simulink model "IP_SwingUp_Design21"  (R2021a)
settings: Solver=VariableStepAuto  StartTime=0.0  StopTime=30  FixedStep=0.01  RelTol=1e-3
values from neighbouring files (symbols this model uses):
  b = 0.0    (= 0)    [Init_Setup_LQRArd.m]
  c = 1.5    [Init_Setup_LQRArd.m]
  Er = 2*m*g*l    (= 0.36113784)    [Init_Setup_LQRArd.m]
  g = 9.8    [Init_Setup_LQRArd.m]
  I = 0.00527    [Init_Setup_LQRArd.m]
  l = 0.26322    [Init_Setup_LQRArd.m]
  M = 0.25    [Init_Setup_LQRArd.m]
  m = 0.07    [Init_Setup_LQRArd.m]
  M_c = 0.25    [Init_Setup_LQRArd.m]
  n = 1.05    [Init_Setup_LQRArd.m]
libraries: simulink x4
settings Model: Creator=jitendra  LastModifiedBy=M7540
settings SolverCC: AlgebraicLoopSolver=LineSearch
settings DataIOCC: ExternalInput=getinputstruct(op_trim1)  InitialState=getstatestruct(op_trim1)  ReturnWorkspaceOutputs=off
settings DebuggingCC: SFMachineParentedDataDiag=warning  ArithmeticOperatorsInVariantConditions=warning
settings SFSimCC: SimUseLocalCustomCode=off  CustomCodeUndefinedFunction=UseInterfaceOnly
settings RTWCC: RTWUseLocalCustomCode=off

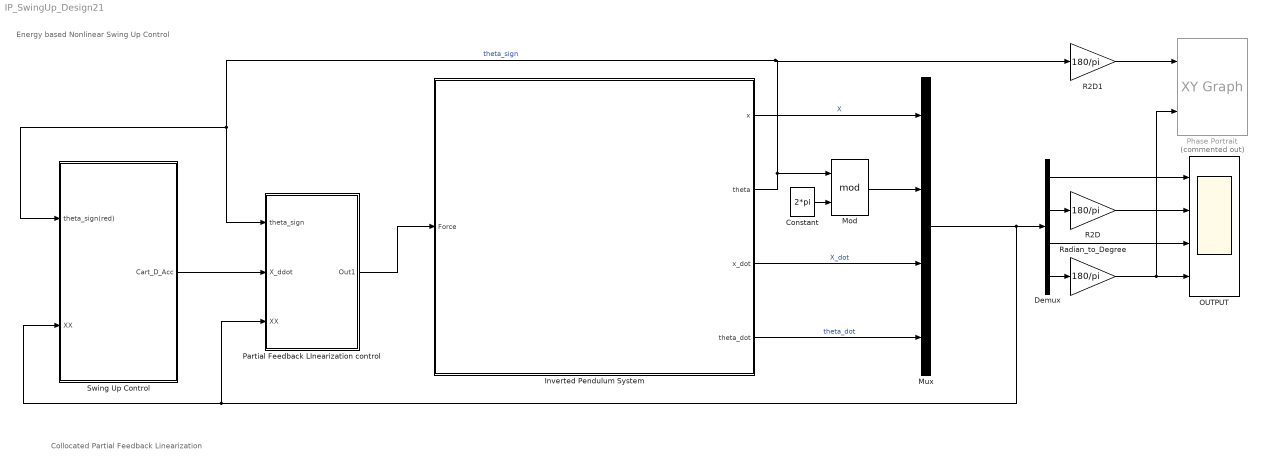
== system IP_SwingUp_Design21 ==
  note: Collocated Partial
      | Feedback Linearization
  note: Energy based
      | Nonlinear
      | Swing Up Control
  Constant : Constant  Value=2*pi
  Demux : Demux
  Inverted Pendulum System : Subsystem
      mask Display: image('ip_model.png');
  Mod : Math  Operator=mod  SignedPower=on  SaturateOnIntegerOverflow=on
  Mux : Mux
  OUTPUT : Scope  NumInputPorts=4
  Partial Feedback LInearization control : Subsystem
  Phase Portrait : simulink/Sinks/XY Graph  Commented=on  xmin=-190  xmax=200  ymin=-700  ymax=700  st=-1
  R2D : Gain  Gain=180/pi
  R2D1 : Gain  Gain=180/pi
  Radian_to_Degree : Gain  Gain=180/pi
  Swing Up Control : Subsystem
  wires:
  Inverted Pendulum System/3(x_dot) -> Mux/3  "X_dot"
  Inverted Pendulum System/1(x) -> Mux/1  "X"
  Inverted Pendulum System/4(theta_dot) -> Mux/4  "theta_dot"
  Mux/1 -> Demux/1, Swing Up Control/2(XX), Partial Feedback LInearization control/3(XX)
  Demux/2 -> R2D/1
  Demux/1 -> OUTPUT/1
  Demux/3 -> OUTPUT/3
  Demux/4 -> Radian_to_Degree/1
  R2D/1 -> OUTPUT/2
  Swing Up Control/1(Cart_D_Acc) -> Partial Feedback LInearization control/2(X_ddot)
  Constant/1 -> Mod/2
  Inverted Pendulum System/2(theta) -> R2D1/1, Partial Feedback LInearization control/1(theta_sign), Swing Up Control/1(theta_sign(red)), Mod/1  "theta_sign"
  Mod/1 -> Mux/2
  Radian_to_Degree/1 -> Phase Portrait/2, OUTPUT/4
  R2D1/1 -> Phase Portrait/1
  Partial Feedback LInearization control/1(Out1) -> Inverted Pendulum System/1(Force)

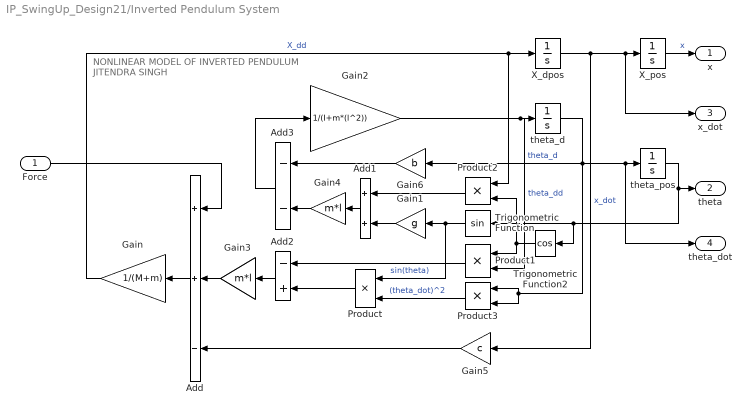
== system IP_SwingUp_Design21/Inverted Pendulum System ==
  note: NONLINEAR MODEL OF
      | INVERTED PENDULUM
      | JITENDRA SINGH
  Force : Inport
  Add : Sum  Inputs=++-
  Add1 : Sum
  Add2 : Sum  Inputs=-+
  Add3 : Sum  Inputs=--
  Gain : Gain  Gain=1/(M+m)
  Gain1 : Gain  Gain=g
  Gain2 : Gain  Gain=1/(I+m*(l^2))
  Gain3 : Gain  Gain=m*l
  Gain4 : Gain  Gain=m*l
  Gain5 : Gain  Gain=c
  Gain6 : Gain  Gain=b
  Product{,1..3} (4 alike) : Product
  Trigonometric Function : Trigonometry
  Trigonometric Function2 : Trigonometry  Operator=cos
  X_dpos : Integrator
  X_pos : Integrator
  theta_d : Integrator
  theta_pos : Integrator  InitialCondition=1*(pi/180)
  x : Outport  VectorParamsAs1DForOutWhenUnconnected=off
  theta : Outport  Port=2  VectorParamsAs1DForOutWhenUnconnected=off
  x_dot : Outport  Port=3  VectorParamsAs1DForOutWhenUnconnected=off
  theta_dot : Outport  Port=4  VectorParamsAs1DForOutWhenUnconnected=off
  wires:
  Gain5/1 -> Add/3
  Add2/1 -> Gain3/1
  Add3/1 -> Gain2/1
  Trigonometric Function2/1 -> Product2/2, Product1/1
  Trigonometric Function/1 -> Product/1, Gain1/1  "sin(theta)"
  Gain3/1 -> Add/2
  theta_d/1 -> Product3/2, Product3/1, Gain6/1, theta_dot/1, theta_pos/1  "theta_d"
  Product2/1 -> Add1/1
  Product/1 -> Add2/2
  Gain4/1 -> Add3/2
  Product3/1 -> Product/2  "(theta_dot)^2"
  X_pos/1 -> x/1  "x"
  Product1/1 -> Add2/1
  Gain/1 -> X_dpos/1, Product2/1  "X_dd"
  Add/1 -> Gain/1
  Gain2/1 -> Product1/2, theta_d/1  "theta_dd"
  Gain6/1 -> Add3/1
  theta_pos/1 -> Trigonometric Function2/1, Trigonometric Function/1, theta/1
  Force/1 -> Add/1
  Gain1/1 -> Add1/2
  X_dpos/1 -> x_dot/1, X_pos/1, Gain5/1  "x_dot"
  Add1/1 -> Gain4/1

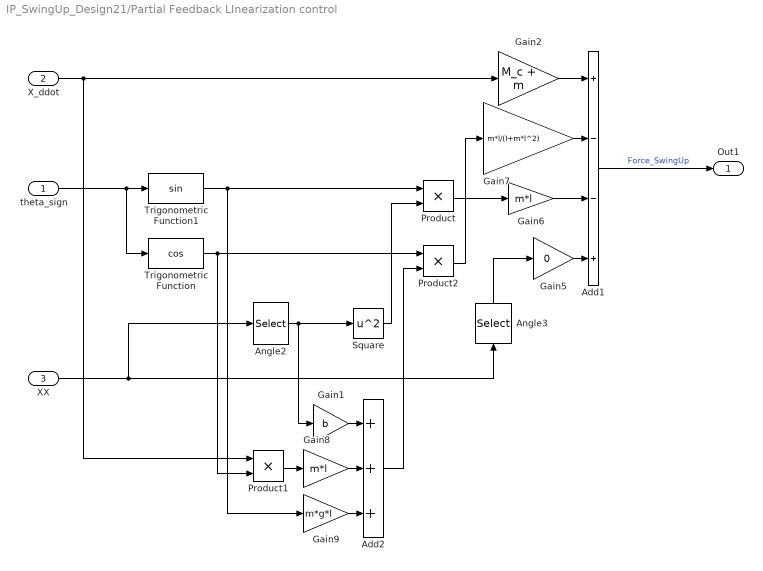
== system IP_SwingUp_Design21/Partial Feedback LInearization control ==
  theta_sign : Inport
  X_ddot : Inport  Port=2
  XX : Inport  Port=3
  Add1 : Sum  Inputs=+--+
  Add2 : Sum  Inputs=+++
  Angle2 : Selector  InputPortWidth=4  IndexOptions=Index vector (dialog)  Indices=[4]  OutputSizes=1
  Angle3 : Selector  InputPortWidth=4  IndexOptions=Index vector (dialog)  Indices=[3]  OutputSizes=1
  Gain1 : Gain  Gain=b
  Gain2 : Gain  Gain=M_c + m
  Gain5 : Gain  Gain=0
  Gain6 : Gain  Gain=m*l
  Gain7 : Gain  Gain=m*l/(I+m*l^2)
  Gain8 : Gain  Gain=m*l
  Gain9 : Gain  Gain=m*g*l
  Product : Product
  Product1 : Product
  Product2 : Product
  Square : Math  Operator=square  SignedPower=on  RndMeth=Zero  SaturateOnIntegerOverflow=on
  Trigonometric Function : Trigonometry  Operator=cos
  Trigonometric Function1 : Trigonometry
  Out1 : Outport  VectorParamsAs1DForOutWhenUnconnected=off
  wires:
  Angle3/1 -> Gain5/1
  X_ddot/1 -> Gain2/1, Product1/1
  Gain2/1 -> Add1/1
  Add1/1 -> Out1/1  "Force_SwingUp"
  Gain5/1 -> Add1/4
  Gain7/1 -> Add1/2
  theta_sign/1 -> Trigonometric Function/1, Trigonometric Function1/1
  XX/1 -> Angle3/1, Angle2/1
  Angle2/1 -> Square/1, Gain1/1
  Product/1 -> Gain6/1
  Trigonometric Function1/1 -> Product/1, Gain9/1
  Square/1 -> Product/2
  Gain6/1 -> Add1/3
  Gain1/1 -> Add2/1
  Product1/1 -> Gain8/1
  Trigonometric Function/1 -> Product2/1, Product1/2
  Gain8/1 -> Add2/2
  Gain9/1 -> Add2/3
  Add2/1 -> Product2/2
  Product2/1 -> Gain7/1

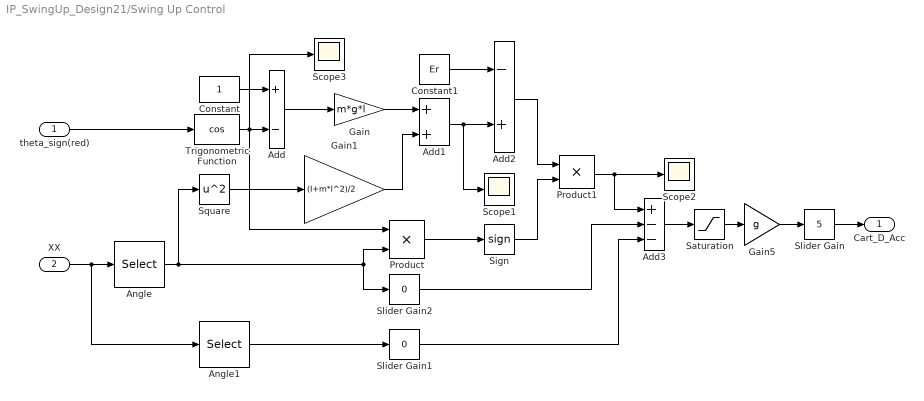
== system IP_SwingUp_Design21/Swing Up Control ==
  theta_sign(red) : Inport
  XX : Inport  Port=2
  Add : Sum  Inputs=+-
  Add1 : Sum
  Add2 : Sum  Inputs=-+
  Add3 : Sum  Inputs=+--
  Angle : Selector  InputPortWidth=4  IndexOptions=Index vector (dialog)  Indices=[4]  OutputSizes=1
  Angle1 : Selector  InputPortWidth=4  IndexOptions=Index vector (dialog)  Indices=[1]  OutputSizes=1
  Constant : Constant
  Constant1 : Constant  Value=Er
  Gain : Gain  Gain=m*g*l
  Gain1 : Gain  Gain=(I+m*l^2)/2
  Gain5 : Gain  Gain=g
  Product : Product
  Product1 : Product
  Saturation : Saturate  UpperLimit=n*g  LowerLimit=-n*g
  Scope1 : Scope
  Scope2 : Scope
  Scope3 : Scope
  Sign : Signum
  Slider Gain : simulink/Math Operations/Slider Gain  gain=5  low=0  high=30
  Slider Gain1 : simulink/Math Operations/Slider Gain  gain=0  low=0  high=5
  Slider Gain2 : simulink/Math Operations/Slider Gain  gain=0  low=0  high=5
  Square : Math  Operator=square  SignedPower=on  RndMeth=Zero  SaturateOnIntegerOverflow=on
  Trigonometric Function : Trigonometry  Operator=cos
  Cart_D_Acc : Outport  VectorParamsAs1DForOutWhenUnconnected=off
  wires:
  Constant/1 -> Add/1
  Add/1 -> Gain/1
  Trigonometric Function/1 -> Scope3/1, Product/1, Add/2
  Square/1 -> Gain1/1
  XX/1 -> Angle1/1, Angle/1
  Gain/1 -> Add1/1
  Gain1/1 -> Add1/2
  Product/1 -> Sign/1
  Add1/1 -> Scope1/1, Add2/2
  Add2/1 -> Product1/1
  Sign/1 -> Product1/2
  Product1/1 -> Scope2/1, Add3/1
  Saturation/1 -> Gain5/1
  Slider Gain/1 -> Cart_D_Acc/1
  Gain5/1 -> Slider Gain/1
  theta_sign(red)/1 -> Trigonometric Function/1
  Constant1/1 -> Add2/1
  Angle/1 -> Slider Gain2/1, Product/2, Square/1
  Angle1/1 -> Slider Gain1/1
  Slider Gain2/1 -> Add3/2
  Slider Gain1/1 -> Add3/3
  Add3/1 -> Saturation/1
